simulink model "Triple_rotor_Tilerotor_model"  (R2024b)
settings: Solver=ode45  StartTime=0.0  StopTime=100  FixedStep=1e-3  RelTol=1e-3
values from neighbouring files (symbols this model uses):
  para =     [Triple_Rotors_Tilrotor_Parameters.mat]
undefined symbols (not defined in the file or in its folder): initial_height, initial_pitch, initial_vx, magnitude, rot2
libraries: simulink x9, slpidlib x5, matrix_library x4, vrlib x1
(part 3 of 3)

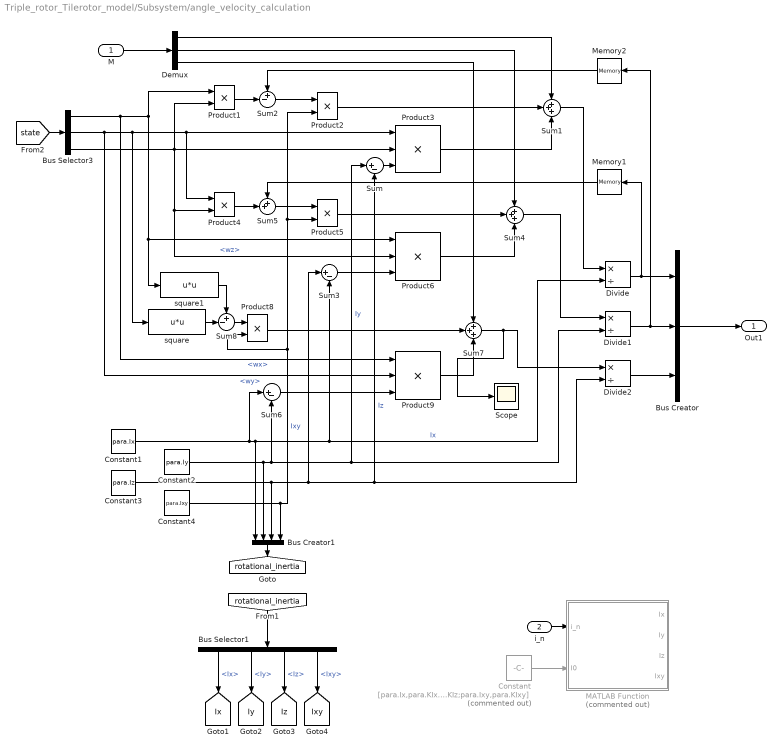
== system Triple_rotor_Tilerotor_model/Subsystem/angle_velocity_calculation ==
  M : Inport
  i_n : Inport  Port=2
  Bus Creator : BusCreator  Inputs=3
  Bus Creator1 : BusCreator  Inputs=4
  Bus Selector1 : BusSelector  OutputSignals=Ix,Iy,Iz,Ixy
  Bus Selector3 : BusSelector  OutputSignals=wx,wy,wz
  Constant : Constant  Commented=on  Value=[para.Ix,para.KIx;para.Iy,para.KIy;para.Iz,para.KIz;para.Ixy,para.KIxy]
  Constant1 : Constant  Value=para.Ix
  Constant2 : Constant  Value=para.Iy
  Constant3 : Constant  Value=para.Iz
  Constant4 : Constant  Value=para.Ixy
  Demux : Demux  Outputs=3
  Divide : Product  Inputs=*/
  Divide1 : Product  Inputs=*/
  Divide2 : Product  Inputs=*/
  MATLAB Function : MATLAB Function  Commented=on  TreatAsAtomicUnit=on
  Memory1 : Memory
  Memory2 : Memory
  Product{1..2,4..5,8} (5 alike) : Product
  Product3 : Product  Inputs=3
  Product6 : Product  Inputs=3
  Product9 : Product  Inputs=3
  Scope : Scope
  Sum : Sum  Inputs=|+-
  Sum1 : Sum  Inputs=+++
  Sum2 : Sum  Inputs=+-|
  Sum3 : Sum  Inputs=|+-
  Sum4 : Sum  Inputs=+++
  Sum5 : Sum  Inputs=++|
  Sum6 : Sum  Inputs=|+-
  Sum7 : Sum  Inputs=+++
  Sum8 : Sum  Inputs=+-|
  square : MATLABFcn  MATLABFcn=u*u
  square1 : MATLABFcn  MATLABFcn=u*u
  Out1 : Outport
  tag scope: Ix=global, Ixy=global, Iy=global, Iz=global, rotational_inertia=global
  wires:
  Constant3/1 -> Bus Creator1/3, Sum3/1, Divide2/2, Sum/2  "Iz"
  Divide/1 -> Bus Creator/1, Memory1/1
  Constant1/1 -> Bus Creator1/1, Divide/2, Sum3/2, Sum6/1  "Ix"
  Sum7/1 -> Scope/1, Divide2/1
  Constant4/1 -> Bus Creator1/4, Product8/2, Product5/2, Product2/2  "Ixy"
  Sum1/1 -> Divide/1
  Divide2/1 -> Bus Creator/3
  Bus Creator/1 -> Out1/1
  [state] -> Bus Selector3/1
  Bus Selector3/1 -> Product9/1, Product1/1, square1/1, Product6/1  "<wx>"
  Bus Selector3/2 -> Product9/2, square/1, Product4/1, Product3/1  "<wy>"
  Bus Selector3/3 -> Product1/2, Product3/2, Product6/2, Product4/2  "<wz>"
  Constant2/1 -> Bus Creator1/2, Sum6/2, Divide1/2, Sum/1  "Iy"
  Sum/1 -> Product3/3
  M/1 -> Demux/1
  Demux/1 -> Sum1/1
  Product3/1 -> Sum1/3
  Product1/1 -> Sum2/2
  Sum2/1 -> Product2/1
  Product2/1 -> Sum1/2
  Sum5/1 -> Product5/1
  Product6/1 -> Sum4/3
  Sum3/1 -> Product6/3
  Product5/1 -> Sum4/2
  Product4/1 -> Sum5/2
  Demux/2 -> Sum4/1
  Sum8/1 -> Product8/1
  Product9/1 -> Sum7/3
  Sum6/1 -> Product9/3
  Product8/1 -> Sum7/2
  Sum4/1 -> Divide1/1
  square/1 -> Sum8/2
  square1/1 -> Sum8/1
  Demux/3 -> Sum7/1
  Bus Creator1/1 -> [rotational_inertia]
  Divide1/1 -> Memory2/1, Bus Creator/2
  Memory1/1 -> Sum5/1
  Memory2/1 -> Sum2/1
  Bus Selector1/2 -> [Iy]  "<Iy>"
  [rotational_inertia] -> Bus Selector1/1
  Bus Selector1/3 -> [Iz]  "<Iz>"
  Bus Selector1/1 -> [Ix]  "<Ix>"
  Bus Selector1/4 -> [Ixy]  "<Ixy>"
  Constant/1 -> MATLAB Function/2(I0)
  i_n/1 -> MATLAB Function/1(i_n)

== system Triple_rotor_Tilerotor_model/Subsystem/velocity_calculation ==
  F : Inport
  Bus Creator1 : BusCreator  Inputs=3
  Bus Creator2 : BusCreator  Inputs=3
  Bus Selector1 : BusSelector  OutputSignals=vx,vy,vz,wx,wy,wz
  Bus Selector2 : BusSelector  OutputSignals=gamma,psi,theta
  Constant : Constant  Value=para.g * [0; -1; 0]
  Cross Product : vrlib/Utilities/Cross Product
  Earth_to_Body : MATLAB Function  TreatAsAtomicUnit=on
  Gain : Gain  Gain=1/para.m
  Product : Product  Multiplication=Matrix(*)
  Sum : Sum  Inputs=+++
  dv : Outport
  tag scope: Transform_matrix=global
  wires:
  Earth_to_Body/1(R) -> [Transform_matrix]
  Constant/1 -> Product/2
  [state] -> Bus Selector2/1, Bus Selector1/1
  Cross Product/1 -> Sum/1
  Bus Creator1/1 -> Cross Product/2  "w"
  Sum/1 -> dv/1
  Bus Selector1/5 -> Bus Creator1/2  "<wy>"
  Gain/1 -> Sum/2
  Bus Selector2/3 -> Earth_to_Body/3(theta)  "<theta>"
  Bus Creator2/1 -> Cross Product/1  "v"
  Bus Selector2/1 -> Earth_to_Body/1(gamma)  "<gamma>"
  [Transform_matrix] -> Product/1
  Bus Selector1/2 -> Bus Creator2/2  "<vy>"
  Bus Selector1/4 -> Bus Creator1/1  "<wx>"
  Bus Selector1/1 -> Bus Creator2/1  "<vx>"
  Bus Selector1/3 -> Bus Creator2/3  "<vz>"
  Bus Selector2/2 -> Earth_to_Body/2(psi)  "<psi>"
  Product/1 -> Sum/3
  Bus Selector1/6 -> Bus Creator1/3  "<wz>"
  F/1 -> Gain/1

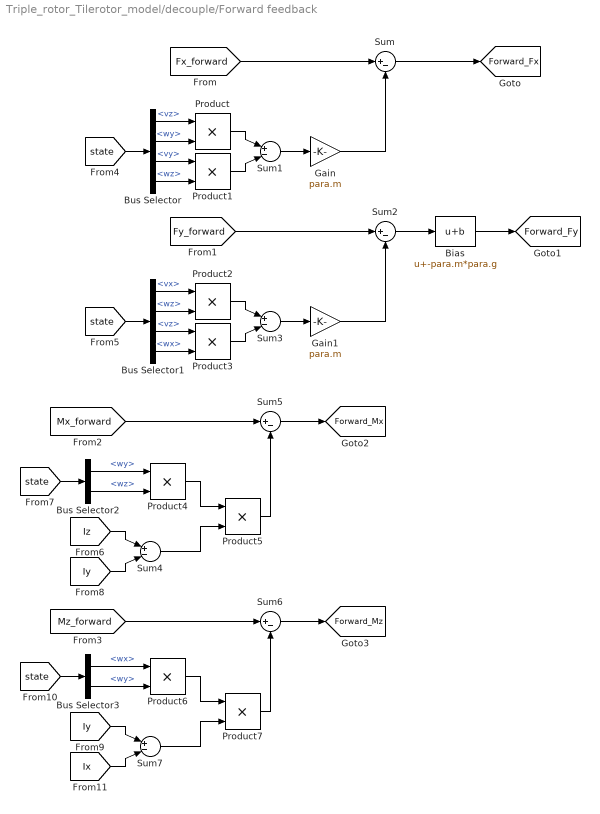
== system Triple_rotor_Tilerotor_model/decouple/Forward feedback ==
  Bias : Bias  Bias=-para.m*para.g  SaturateOnIntegerOverflow=off
  Bus Selector : BusSelector  OutputSignals=vz,wy,vy,wz
  Bus Selector1 : BusSelector  OutputSignals=vx,wz,vz,wx
  Bus Selector2 : BusSelector  OutputSignals=wy,wz
  Bus Selector3 : BusSelector  OutputSignals=wx,wy
  Gain : Gain  Gain=para.m
  Gain1 : Gain  Gain=para.m
  Product{,1..7} (8 alike) : Product
  Sum{,2,5..6} (4 alike) : Sum  Inputs=|+-
  Sum{1,3..4,7} (4 alike) : Sum  Inputs=|+-|
  tag scope: Forward_Fx=global, Forward_Fy=global, Forward_Mx=global, Forward_Mz=global
  wires:
  [Fx_forward] -> Sum/1
  [state] -> Bus Selector/1
  Bus Selector/1 -> Product/1  "<vz>"
  Bus Selector/2 -> Product/2  "<wy>"
  Bus Selector/3 -> Product1/1  "<vy>"
  Bus Selector/4 -> Product1/2  "<wz>"
  Product/1 -> Sum1/1
  Product1/1 -> Sum1/2
  Sum1/1 -> Gain/1
  Gain/1 -> Sum/2
  Sum/1 -> [Forward_Fx]
  [Fy_forward] -> Sum2/1
  Product2/1 -> Sum3/1
  Product3/1 -> Sum3/2
  Bus Selector1/3 -> Product3/1  "<vz>"
  [state] -> Bus Selector1/1
  Gain1/1 -> Sum2/2
  Sum3/1 -> Gain1/1
  Bus Selector1/4 -> Product3/2  "<wx>"
  Bus Selector1/1 -> Product2/1  "<vx>"
  Bus Selector1/2 -> Product2/2  "<wz>"
  Sum2/1 -> Bias/1
  Bias/1 -> [Forward_Fy]
  Bus Selector2/1 -> Product4/1  "<wy>"
  [state] -> Bus Selector2/1
  Bus Selector2/2 -> Product4/2  "<wz>"
  [Iz] -> Sum4/1
  [Iy] -> Sum4/2
  Product4/1 -> Product5/1
  Sum4/1 -> Product5/2
  [Mx_forward] -> Sum5/1
  Product5/1 -> Sum5/2
  Sum5/1 -> [Forward_Mx]
  Sum6/1 -> [Forward_Mz]
  [Mz_forward] -> Sum6/1
  Sum7/1 -> Product7/2
  [Iy] -> Sum7/1
  [state] -> Bus Selector3/1
  Product6/1 -> Product7/1
  [Ix] -> Sum7/2
  Product7/1 -> Sum6/2
  Bus Selector3/1 -> Product6/1  "<wx>"
  Bus Selector3/2 -> Product6/2  "<wy>"

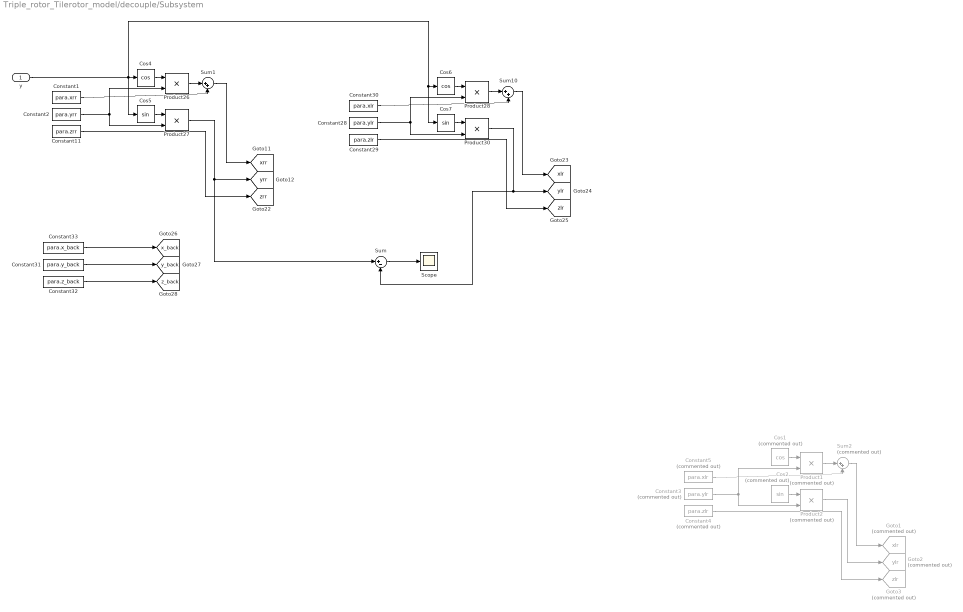
== system Triple_rotor_Tilerotor_model/decouple/Subsystem ==
  y : Inport
  Constant1 : Constant  Value=para.xrr
  Constant11 : Constant  Value=para.zrr
  Constant2 : Constant  Value=para.yrr
  Constant28 : Constant  Value=para.ylr
  Constant29 : Constant  Value=para.zlr
  Constant3 : Constant  Commented=on  Value=para.ylr
  Constant30 : Constant  Value=para.xlr
  Constant31 : Constant  Value=para.y_back
  Constant32 : Constant  Value=para.z_back
  Constant33 : Constant  Value=para.x_back
  Constant4 : Constant  Commented=on  Value=para.zlr
  Constant5 : Constant  Commented=on  Value=para.xlr
  Cos1 : Trigonometry  Commented=on  Operator=cos
  Cos2 : Trigonometry  Commented=on
  Cos4 : Trigonometry  Operator=cos
  Cos5 : Trigonometry
  Cos6 : Trigonometry  Operator=cos
  Cos7 : Trigonometry
  Goto1 : Goto  Commented=on  GotoTag=xlr  TagVisibility=global
  Goto2 : Goto  Commented=on  GotoTag=ylr  TagVisibility=global
  Goto3 : Goto  Commented=on  GotoTag=zlr  TagVisibility=global
  Product1 : Product  Commented=on
  Product2 : Product  Commented=on
  Product{26..28,30} (4 alike) : Product
  Scope : Scope
  Sum : Sum  Inputs=|+-
  Sum1 : Sum  Inputs=|++
  Sum10 : Sum  Inputs=|++
  Sum2 : Sum  Commented=on  Inputs=|++
  tag scope: x_back=global, xlr=global, xrr=global, y_back=global, ylr=global, yrr=global, z_back=global, zlr=global, zrr=global
  wires:
  Constant30/1 -> Sum10/2
  Product28/1 -> Sum10/1
  y/1 -> Cos4/1, Cos7/1, Cos6/1, Cos5/1
  Sum10/1 -> [xlr]
  Constant1/1 -> Sum1/2
  Cos6/1 -> Product28/1
  Constant29/1 -> [zlr]
  Product30/1 -> [ylr], Sum/2
  Constant2/1 -> Product26/2, Product27/2
  Constant11/1 -> [zrr]
  Cos4/1 -> Product26/1
  Constant32/1 -> [z_back]
  Product26/1 -> Sum1/1
  Product27/1 -> Sum/1, [yrr]
  Cos5/1 -> Product27/1
  Constant31/1 -> [y_back]
  Constant28/1 -> Product28/2, Product30/2
  Constant33/1 -> [x_back]
  Cos7/1 -> Product30/1
  Constant3/1 -> Product1/2, Product2/2
  Constant5/1 -> Sum2/2
  Cos2/1 -> Product2/1
  Constant4/1 -> Goto3/1
  Cos1/1 -> Product1/1
  Product2/1 -> Goto2/1
  ? -> Cos2/1, Cos1/1
  Product1/1 -> Sum2/1
  Sum2/1 -> Goto1/1
  Sum/1 -> Scope/1
  Sum1/1 -> [xrr]

== matlab function Triple_rotor_Tilerotor_model/Rotors_dynamic/locate_matrix4 ==
  data: x_back input; R output; y_back input; z_back input
function R = fcn(x_back, y_back, z_back)
% input : 发动机短舱位置坐标
% output : R
% H to Body

R = zeros(3,3);
 
R = [0, z_back, -y_back;...
    -z_back, 0, x_back;...
    y_back, -x_back, 0];

== matlab function Triple_rotor_Tilerotor_model/Rotors_dynamic/locate_matrix5 ==
  data: x_back input; R output; y_back input; z_back input
function R = fcn(x_back, y_back, z_back)
% input : 发动机短舱位置坐标
% output : R
% H to Body

R = zeros(3,3);
 
R = [0, -z_back, y_back;...
    z_back, 0, -x_back;...
    -y_back, x_back, 0];

== matlab function Triple_rotor_Tilerotor_model/Subsystem/velocity_calculation/Earth_to_Body ==
  data: gamma input; R output; psi input; theta input
function R = fcn(gamma,psi,theta)

%earth to body

R = zeros(3,3);
 
R = [cos(psi)*cos(theta)                                 sin(theta)             -sin(psi)*cos(theta);
     -cos(gamma)*cos(psi)*sin(theta)+sin(gamma)*sin(psi) cos(gamma)*cos(theta)  cos(gamma)*sin(psi)*sin(theta)+sin(gamma)*cos(psi);
     sin(gamma)*cos(psi)*sin(theta)+cos(gamma)*sin(psi)  -sin(gamma)*cos(theta) -sin(gamma)*sin(psi)*sin(theta)+cos(gamma)*cos(psi)];

== matlab function Triple_rotor_Tilerotor_model/decouple/acos ==
  data: u input; y output; v input
function y = fcn(u,v)
y = acos( u / sqrt( power(u , 2) + power(v , 2) ));

== matlab function Triple_rotor_Tilerotor_model/Rotors_dynamic/H_to_Body1 ==
  data: i_n input; R output
function R = fcn(i_n)
% input : 旋翼倾转角i_n
% output : R
% H to Body

R = zeros(3,3);
 
R = [sin(i_n), cos(i_n), 0;...
    -cos(i_n), sin(i_n), 0;...
    0, 0, 1];

== matlab function Triple_rotor_Tilerotor_model/Rotors_dynamic/locate_matrix7 ==
  data: xlr input; R output; ylr input; zlr input
function R = fcn(xlr, ylr, zlr)
% input : 发动机短舱位置坐标
% output : R
% H to Body

R = zeros(3,3);
 
R = [0, -zlr, ylr;...
    zlr, 0, -xlr;...
    -ylr, xlr, 0];

== matlab function Triple_rotor_Tilerotor_model/Rotors_dynamic/locate_matrix6 ==
  data: xlr input; R output; ylr input; zlr input
function R = fcn(xlr, ylr, zlr)
% input : 发动机短舱位置坐标
% output : R
% H to Body

R = zeros(3,3);
 
R = [0, zlr, -ylr;...
    -zlr, 0, xlr;...
    ylr, -xlr, 0];

== matlab function Triple_rotor_Tilerotor_model/Rotors_dynamic/H_to_Body3 ==
  data: i_n input; R output
function R = fcn(i_n)
% input : 旋翼倾转角i_n
% output : R
% H to Body

R = zeros(3,3);
 
R = [sin(i_n), cos(i_n), 0;...
    -cos(i_n), sin(i_n), 0;...
    0, 0, 1];

== matlab function Triple_rotor_Tilerotor_model/Rotors_dynamic/H_to_Body_inv ==
  data: i_n input; R output
function R = fcn(i_n)
% input : 旋翼倾转角i_n
% output : R
% H to Body

R = zeros(3,3);
 
R = [sin(i_n), cos(i_n), 0;...
    -cos(i_n), sin(i_n), 0;...
    0, 0, 1];
R = inv(R);

== matlab function Triple_rotor_Tilerotor_model/Rotors_dynamic/H_to_Body_inv1 ==
  data: i_n input; R output
function R = fcn(i_n)
% input : 旋翼倾转角i_n
% output : R
% H to Body

R = zeros(3,3);
 
R = [sin(i_n), cos(i_n), 0;...
    -cos(i_n), sin(i_n), 0;...
    0, 0, 1];
R = inv(R);

== matlab function Triple_rotor_Tilerotor_model/Rotors_dynamic/locate_matrix ==
  data: xrr input; R output; yrr input; zrr input
function R = fcn(xrr, yrr, zrr)
% input : 发动机短舱位置坐标
% output : R
% H to Body

R = zeros(3,3);
 
R = [0, zrr, -yrr;...
    -zrr, 0, xrr;...
    yrr, -xrr, 0];

== matlab function Triple_rotor_Tilerotor_model/Rotors_dynamic/H_to_Body_inv2 ==
  data: i_n input; R output
function R = fcn(i_n)
% input : 旋翼倾转角i_n
% output : R
% H to Body

R = zeros(3,3);
 
R = [sin(i_n), cos(i_n), 0;...
    -cos(i_n), sin(i_n), 0;...
    0, 0, 1];
R = inv(R);

== matlab function Triple_rotor_Tilerotor_model/Rotors_dynamic/locate_matrix1 ==
  data: xrr input; R output; yrr input; zrr input
function R = fcn(xrr, yrr, zrr)
% input : 发动机短舱位置坐标
% output : R
% H to Body

R = zeros(3,3);
 
R = [0, -zrr, yrr;...
    zrr, 0, -xrr;...
    -yrr, xrr, 0];

== matlab function Triple_rotor_Tilerotor_model/Subsystem/angle_velocity_calculation/MATLAB Function ==
  data: i_n input; Ix output; Iy output; Iz output; Ixy output; I0 input
function [Ix, Iy, Iz, Ixy] = fcn(i_n, I0)

Ix = I0(1,1) + I0(1,2)*( - abs(i_n - 90) );%Ix = I0(1,1) + I0(1,2)*(i_n - 90)
Iy = I0(2,1) + I0(2,2)*( - abs(i_n - 90) );%Iy = I0(2,1) + I0(2,2)*(i_n - 90)
Iz = I0(3,1) + I0(3,2)*( - abs(i_n - 90) );
Ixy = I0(4,1) + I0(4,2)*( - abs(i_n - 90) );

== matlab function Triple_rotor_Tilerotor_model/Rotors_dynamic/locate_matrix3 ==
  data: xlr input; R output; ylr input; zlr input
function R = fcn(xlr, ylr, zlr)
% input : 发动机短舱位置坐标
% output : R
% H to Body

R = zeros(3,3);
 
R = [0, zlr, -ylr;...
    -zlr, 0, xlr;...
    ylr, -xlr, 0];
